simulink model "Practica_5_slx"  (R2023b)
settings: Solver=ode4  StartTime=0.0  StopTime=3000  FixedStep=0.01  RelTol=1e-3
values from neighbouring files (symbols this model uses):
  Qi = 8 / (1000*60)    (= 0.000133333333333)    [Practica_5.m]
  ue = Qi / (Ao*sqrt(2*g*x1e))    [Practica_5.m]
  x1e = 0.45    [Practica_5.m]
  ye = x1e    (= 0.45)    [Practica_5.m]
libraries: cstblocks x5
settings Model: Creator=aghersin  LastModifiedBy=Zoe
settings SolverCC: AlgebraicLoopSolver=TrustRegion
settings DataIOCC: ReturnWorkspaceOutputs=off
settings OptimizationCC: LifeSpan=inf
settings DebuggingCC: UnconnectedInputMsg=warning  UnconnectedOutputMsg=warning  UnconnectedLineMsg=warning  SFExecutionAtInitializationDiag=none  ArithmeticOperatorsInVariantConditions=warning
settings ModelReferenceCC: EnableRefExpFcnMdlSchedulingChecks=on
settings SFSimCC: SimUseLocalCustomCode=off  CustomCodeUndefinedFunction=UseInterfaceOnly
settings RTWCC: RTWUseLocalCustomCode=off
settings CodeAppCC: StateflowObjectComments=on

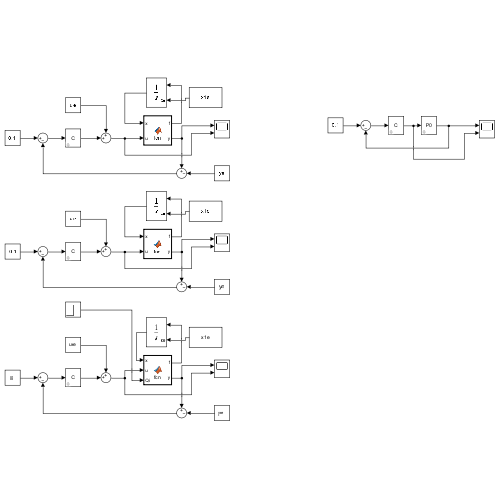
[thumbnail: Simulink's stored preview of the top-level diagram]
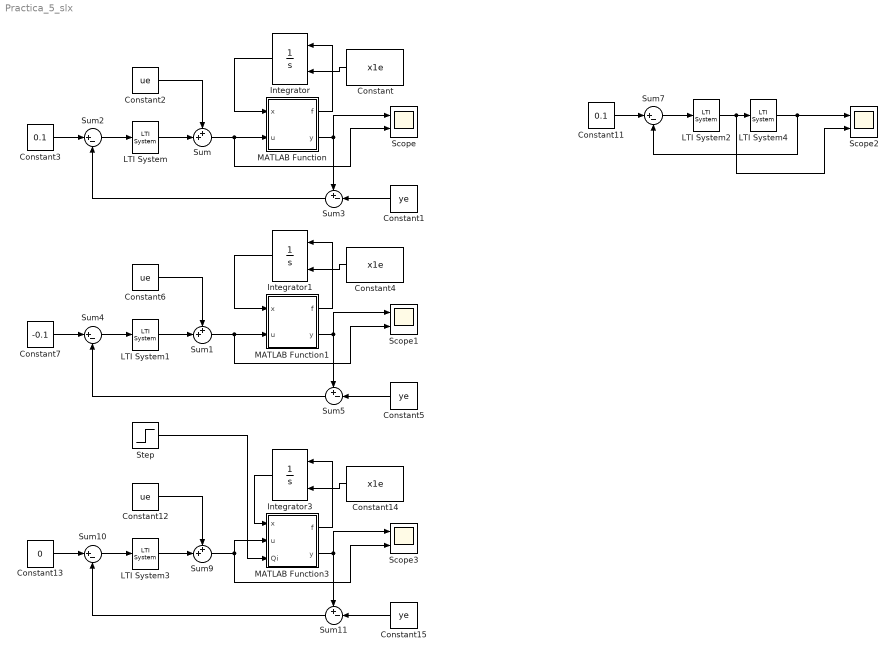
== system Practica_5_slx ==
  Constant : Constant  Value=x1e
  Constant1 : Constant  Value=ye
  Constant11 : Constant  Value=0.1
  Constant12 : Constant  Value=ue
  Constant13 : Constant  Value=0
  Constant14 : Constant  Value=x1e
  Constant15 : Constant  Value=ye
  Constant2 : Constant  Value=ue
  Constant3 : Constant  Value=0.1
  Constant4 : Constant  Value=x1e
  Constant5 : Constant  Value=ye
  Constant6 : Constant  Value=ue
  Constant7 : Constant  Value=-0.1
  Integrator : Integrator  InitialConditionSource=external
  Integrator1 : Integrator  InitialConditionSource=external
  Integrator3 : Integrator  InitialConditionSource=external
  LTI System{,1..3} (4 alike) : cstblocks/LTI System  sys=C  IC=[]  PadeOrder=0
  LTI System4 : cstblocks/LTI System  sys=P0  IC=[]  PadeOrder=0
  MATLAB Function : MATLAB Function  TreatAsAtomicUnit=on
  MATLAB Function1 : MATLAB Function  TreatAsAtomicUnit=on
  MATLAB Function3 : MATLAB Function  TreatAsAtomicUnit=on
  Scope{,1..3} (4 alike) : Scope  NumInputPorts=2
  Step : Step  Time=100  Before=Qi  After=Qi*1.1  SampleTime=0
  Sum : Sum  Inputs=++|
  Sum1 : Sum  Inputs=++|
  Sum{2,4,7,10} (4 alike) : Sum  Inputs=|+-
  Sum11 : Sum  Inputs=+-|
  Sum3 : Sum  Inputs=+-|
  Sum5 : Sum  Inputs=+-|
  Sum9 : Sum  Inputs=++|
  wires:
  Integrator/1 -> MATLAB Function/1(x)
  MATLAB Function/1(f) -> Integrator/1
  Constant/1 -> Integrator/2
  MATLAB Function/2(y) -> Sum3/1, Scope/1
  Constant1/1 -> Sum3/2
  Constant2/1 -> Sum/1
  Sum2/1 -> LTI System/1
  Constant3/1 -> Sum2/1
  Sum3/1 -> Sum2/2
  LTI System/1 -> Sum/2
  Sum/1 -> Scope/2, MATLAB Function/2(u)
  LTI System1/1 -> Sum1/2
  Sum5/1 -> Sum4/2
  Constant7/1 -> Sum4/1
  Sum4/1 -> LTI System1/1
  Constant5/1 -> Sum5/2
  MATLAB Function1/1(f) -> Integrator1/1
  Constant4/1 -> Integrator1/2
  Integrator1/1 -> MATLAB Function1/1(x)
  Sum1/1 -> Scope1/2, MATLAB Function1/2(u)
  MATLAB Function1/2(y) -> Sum5/1, Scope1/1
  Constant6/1 -> Sum1/1
  Constant14/1 -> Integrator3/2
  Constant15/1 -> Sum11/2
  Integrator3/1 -> MATLAB Function3/1(x)
  MATLAB Function3/2(y) -> Sum11/1, Scope3/1
  Sum9/1 -> Scope3/2, MATLAB Function3/2(u)
  MATLAB Function3/1(f) -> Integrator3/1
  Sum11/1 -> Sum10/2
  Sum10/1 -> LTI System3/1
  Constant12/1 -> Sum9/1
  Constant13/1 -> Sum10/1
  LTI System3/1 -> Sum9/2
  Step/1 -> MATLAB Function3/3(Qi)
  Constant11/1 -> Sum7/1
  Sum7/1 -> LTI System2/1
  LTI System2/1 -> Scope2/2, LTI System4/1
  LTI System4/1 -> Scope2/1, Sum7/2

== matlab function Practica_5_slx/MATLAB Function1 ==
  data: x input; u input; f output; y output
function [f,y] = fcn(x,u)

Qi = 8 / (1000*60);
d = 0.01065;
l1 = 0.1;
l2 = 0.4;
L = 0.9;
Ao = pi * (d/2)^2;
g = 9.8;

f = (Qi - Ao*u*sqrt(2*g*x)) / (l1 + (x/L)*(l2-l1))^2;

y = x;

== matlab function Practica_5_slx/MATLAB Function ==
  data: x input; u input; f output; y output
function [f,y] = fcn(x,u)

Qi = 8 / (1000*60);
d = 0.01065;
l1 = 0.1;
l2 = 0.4;
L = 0.9;
Ao = pi * (d/2)^2;
g = 9.8;

f = (Qi - Ao*u*sqrt(2*g*x)) / (l1 + (x/L)*(l2-l1))^2;

y = x;

== matlab function Practica_5_slx/MATLAB Function3 ==
  data: x input; u input; f output; y output; Qi input
function [f,y] = fcn(x,u, Qi)

d = 0.01065;
l1 = 0.1;
l2 = 0.4;
L = 0.9;
Ao = pi * (d/2)^2;
g = 9.8;

f = (Qi - Ao*u*sqrt(2*g*x)) / (l1 + (x/L)*(l2-l1))^2;

y = x;
